simulink model "Application_Software"  (R2020b)
settings: configuration reference "freeConfigSet_Sim_ASW" (kept outside this file)
model workspace (MAT data in the model file):
  TsModel = 0.0005
settings Model: ExtModeTrigDuration=8  Creator=vivekr  LastModifiedBy=vlenzi
settings ConfigSetRef: SourceName=freeConfigSet_Sim_ASW  SourceLocation=Base Workspace

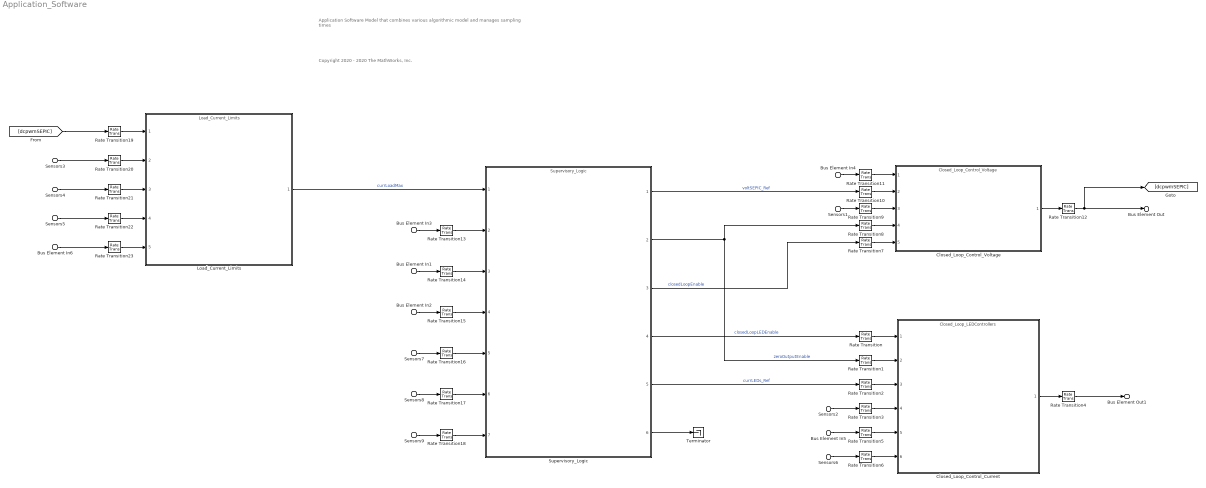
== system Application_Software ==
  note: Application Software
      | Model that combines various algorithmic model and manages sampling times
  note: Copyright 2020 - 2020 The MathWorks, Inc.
  Bus Element In3 : Inport  PortName=UserDefinedValues  Element=voltSEPIC_Desired
  Bus Element In1 : Inport  PortName=UserDefinedValues  Element=currLED_Desired
  Bus Element In2 : Inport  ClipboardFcn=%<Port>  PortName=UserDefinedValues  Element=desiredOperatingMode
  Bus Element In4 : Inport  PortName=UserDefinedValues  Element=dcpwmSEPIC_Desired
  Bus Element In5 : Inport  PortName=UserDefinedValues  Element=dcpwmLED_Desired
  Bus Element In6 : Inport  PortName=UserDefinedValues  Element=currLEDMax_Desired
  Sensors1 : Inport  Port=2  PortName=Sensors  Element=voltSEPIC
  Sensors3 : Inport  Port=2  PortName=Sensors  Element=voltSEPIC
  Sensors6 : Inport  Port=2  PortName=Sensors  Element=voltSEPIC
  Sensors7 : Inport  ClipboardFcn=%<Port>  Port=2  PortName=Sensors  Element=voltSEPIC
  Sensors2 : Inport  Port=2  PortName=Sensors  Element=currLEDstrips
  Sensors4 : Inport  Port=2  PortName=Sensors  Element=currLEDstrips
  Sensors8 : Inport  Port=2  PortName=Sensors  Element=currSEPIC
  Sensors5 : Inport  Port=2  PortName=Sensors  Element=voltPSU
  Sensors9 : Inport  Port=2  PortName=Sensors  Element=voltPSU
  Closed_Loop_Control_Current : ModelReference  ModelNameDialog=Closed_Loop_LEDControllers.slx  SimulationMode=Normal  ModelReferenceVersion=2.16
  Closed_Loop_Control_Voltage : ModelReference  ModelNameDialog=Closed_Loop_Control_Voltage  SimulationMode=Normal  ModelReferenceVersion=2.19
  Load_Current_Limits : ModelReference  ModelNameDialog=Load_Current_Limits  SimulationMode=Normal  ModelReferenceVersion=1.545
  Rate Transition{,1..7,9..12} (12 alike) : RateTransition  Deterministic=off  OutPortSampleTime=ts1ms
  Rate Transition{13..23} (11 alike) : RateTransition
  Rate Transition8 : RateTransition  Deterministic=off  InitialCondition=1  OutPortSampleTime=ts1ms
  Supervisory_Logic : ModelReference  ModelNameDialog=Supervisory_Logic  SimulationMode=Normal  ModelReferenceVersion=1.604
  Terminator : Terminator
  Bus Element Out : Outport  PortName=AppSoftware  Element=dcpwmSEPIC
  Bus Element Out1 : Outport  PortName=AppSoftware  Element=dcpwmLEDvector
  wires:
  Bus Element In2/1 -> Rate Transition15/1
  Closed_Loop_Control_Current/1 -> Rate Transition4/1
  Sensors1/1 -> Rate Transition9/1
  Sensors2/1 -> Rate Transition3/1
  [dcpwmSEPIC] -> Rate Transition19/1
  Sensors3/1 -> Rate Transition20/1
  Sensors4/1 -> Rate Transition21/1
  Sensors5/1 -> Rate Transition22/1
  Bus Element In3/1 -> Rate Transition13/1
  Bus Element In1/1 -> Rate Transition14/1
  Supervisory_Logic/1 -> Rate Transition10/1  "voltSEPIC_Ref"
  Supervisory_Logic/5 -> Rate Transition2/1  "currLEDs_Ref"
  Supervisory_Logic/3 -> Rate Transition7/1  "closedLoopEnable"
  Bus Element In4/1 -> Rate Transition11/1
  Rate Transition/1 -> Closed_Loop_Control_Current/1
  Rate Transition1/1 -> Closed_Loop_Control_Current/2
  Rate Transition2/1 -> Closed_Loop_Control_Current/3
  Rate Transition3/1 -> Closed_Loop_Control_Current/4
  Rate Transition4/1 -> Bus Element Out1/1
  Supervisory_Logic/4 -> Rate Transition/1  "closedLoopLEDEnable"
  Rate Transition5/1 -> Closed_Loop_Control_Current/5
  Bus Element In5/1 -> Rate Transition5/1
  Sensors6/1 -> Rate Transition6/1
  Rate Transition6/1 -> Closed_Loop_Control_Current/6
  Bus Element In6/1 -> Rate Transition23/1
  Sensors7/1 -> Rate Transition16/1
  Sensors8/1 -> Rate Transition17/1
  Sensors9/1 -> Rate Transition18/1
  Supervisory_Logic/2 -> Rate Transition8/1, Rate Transition1/1  "zeroOutputEnable"
  Rate Transition8/1 -> Closed_Loop_Control_Voltage/4
  Rate Transition7/1 -> Closed_Loop_Control_Voltage/5
  Rate Transition9/1 -> Closed_Loop_Control_Voltage/3
  Rate Transition10/1 -> Closed_Loop_Control_Voltage/2
  Rate Transition11/1 -> Closed_Loop_Control_Voltage/1
  Closed_Loop_Control_Voltage/1 -> Rate Transition12/1
  Rate Transition13/1 -> Supervisory_Logic/2
  Rate Transition14/1 -> Supervisory_Logic/3
  Rate Transition15/1 -> Supervisory_Logic/4
  Rate Transition16/1 -> Supervisory_Logic/5
  Rate Transition17/1 -> Supervisory_Logic/6
  Rate Transition18/1 -> Supervisory_Logic/7
  Rate Transition19/1 -> Load_Current_Limits/1
  Rate Transition20/1 -> Load_Current_Limits/2
  Rate Transition21/1 -> Load_Current_Limits/3
  Rate Transition22/1 -> Load_Current_Limits/4
  Rate Transition23/1 -> Load_Current_Limits/5
  Load_Current_Limits/1 -> Supervisory_Logic/1  "currLoadMax"
  Rate Transition12/1 -> [dcpwmSEPIC], Bus Element Out/1
  Supervisory_Logic/6 -> Terminator/1
